simulink model "ADRC"  (R2024b)
settings: Solver=VariableStepAuto  StartTime=0.0  StopTime=40  FixedStep=0.001  RelTol=1e-3  EnableMultiTasking=on
settings Model: TunableVars=PP,PI,PD  TunableVarsStorageClass=ExportedGlobal,ExportedGlobal,ImportedExtern  TunableVarsTypeQualifier=const,const,const  Creator=yuy  LastModifiedBy=17989
settings SolverCC: AlgebraicLoopSolver=TrustRegion
settings DataIOCC: LimitDataPoints=on  SaveFormat=Array  ReturnWorkspaceOutputs=off
settings OptimizationCC: DefaultParameterBehavior=Inlined  LifeSpan=inf
settings DebuggingCC: AlgebraicLoopMsg=none  UnconnectedInputMsg=warning  UnconnectedOutputMsg=warning  UnconnectedLineMsg=warning  SFUnexpectedBacktrackingDiag=warning  SFNoUnconditionalDefaultTransitionDiag=warning  SFExecutionAtInitializationDiag=none  ArithmeticOperatorsInVariantConditions=warning
settings HardwareCC: ProdBitPerPointer=32  ProdBitPerSizeT=32  ProdBitPerPtrDiffT=32  ProdLargestAtomicFloat=None  ProdIntDivRoundTo=Undefined  ProdEndianess=Unspecified  ProdWordSize=32  ProdHWDeviceType=32-bit Generic
settings ModelReferenceCC: EnableRefExpFcnMdlSchedulingChecks=on  PropagateSignalLabelsOutOfModel=off
settings SFSimCC: SimUseLocalCustomCode=off  CustomCodeUndefinedFunction=UseInterfaceOnly
settings RTWCC: GenCodeOnly=on  PackageGeneratedCodeAndArtifacts=on  PackageName=ADRC  RTWUseLocalCustomCode=off  Toolchain=Microsoft Visual C++ 2017 v15.0 | nmake (64-bit Windows)  GPUComputeCapability=3.5
settings CodeAppCC: StateflowObjectComments=on
settings GRTTargetCC: TargetLangStandard=C89/C90 (ANSI)
settings ConfigComp: CovMetricSettings=dw  CovSaveCumulativeToWorkspaceVar=on  CovSaveSingleToWorkspaceVar=on  CovExternalEMLEnable=off  CovSFcnEnable=off

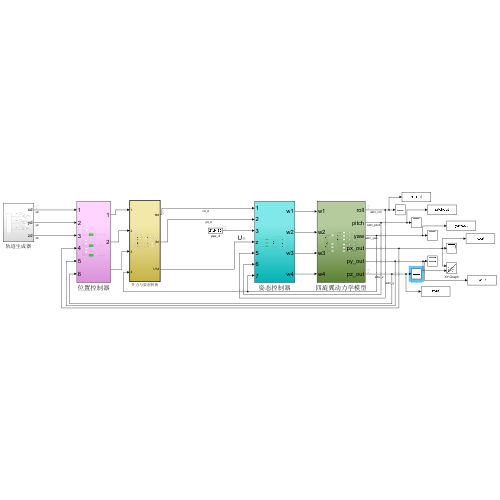
[thumbnail: Simulink's stored preview of the top-level diagram]
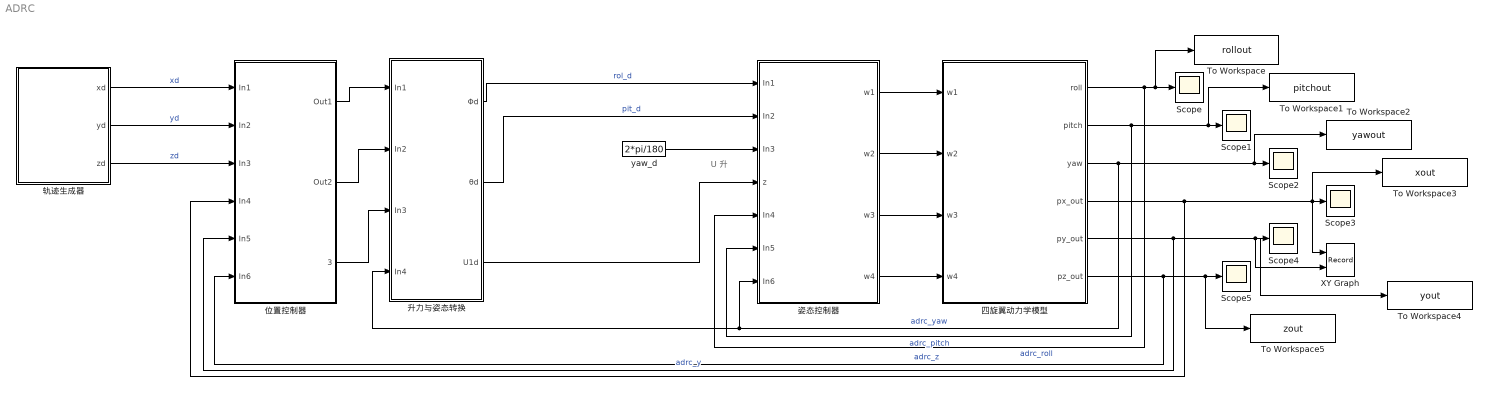
== system ADRC ==
  note: U 升
  Scope{,1..5} (6 alike) : Scope
  To Workspace : ToWorkspace  VariableName=rollout  SampleTime=-1
  To Workspace1 : ToWorkspace  VariableName=pitchout  SampleTime=-1
  To Workspace2 : ToWorkspace  VariableName=yawout  SampleTime=-1
  To Workspace3 : ToWorkspace  VariableName=xout  SampleTime=-1
  To Workspace4 : ToWorkspace  VariableName=yout  SampleTime=-1
  To Workspace5 : ToWorkspace  VariableName=zout  SampleTime=-1
  XY Graph : Record  FileSettingsInternal="{\"entries\":[{\"content\":{\"excelSettings\":{\"content\":{},\"type\":\"Streamout.ExcelSettings\"}},\"type\":\"Streamout.FileSettingStorage\",\"uuid\":\"\"}],\"packageUris\":[\"http:\\/\\/schema.mathworks.com\\/mf0\\/streamout_blocks\\/R2020a\"],\"version\":\"1.0\"}"  Layout=[1 1]  SignalsInternal="{\"entries\":[{\"content\":{\"signals\":[{\"content\":{\"blockPath\":[],\"dimensions\":[1],\"domain\":\"\",\"lineColor\":\"#a2142f\",\"lineWidth\":2,\"port\":1,\"sid\":[\"\"],\"signalID\":1,\"signalName\":\"四旋翼动力学模型:4\"},\"type\":\"RecordBlkView.Signal\",\"uuid\":\"\"},{\"content\":{\"blockPath\":[],\"dimensions\":[1],\"domain\":\"\",\"lineColor\":\"#139fff\",\"lineWidth\":2,\"port\":2,\"sid\":[\"\"],\"signalID\":2,\"signalName\":\"adrc_y\"},\"type\":\"RecordBlkView.Signal\",\"uuid\":\"\"}]},\"type\":\"RecordBlkView.InputSignals\",\"uuid\":\"\"}],\"packageUris\":[\"http:\\/\\/schema.mathworks.com\\/mf0\\/streamout_blocks\\/R2020a\"],\"version\":\"1.0\"}"  VisualizationBindings="{\"xyplotplugin\":{\"info\":[{\"series\":[],\"subplotID\":1}]}}"  CompatibilityTag=XY  st=-1
  yaw_d : Constant  Value=2*pi/180
  位置控制器 : Subsystem
  升力与姿态转换 : Subsystem  TreatAsAtomicUnit=on
  四旋翼动力学模型 : Subsystem
  姿态控制器 : Subsystem
  轨迹生成器 : Subsystem
  wires:
  四旋翼动力学模型/4(px_out) -> To Workspace3/1, XY Graph/1, Scope3/1, 位置控制器/4(In4)
  四旋翼动力学模型/5(py_out) -> To Workspace4/1, XY Graph/2, Scope4/1, 位置控制器/5(In5)  "adrc_y"
  四旋翼动力学模型/6(pz_out) -> To Workspace5/1, Scope5/1, 位置控制器/6(In6)  "adrc_z"
  四旋翼动力学模型/1(roll) -> To Workspace/1, Scope/1, 姿态控制器/5(In4)  "adrc_roll"
  姿态控制器/1(w1) -> 四旋翼动力学模型/1(w1)
  姿态控制器/2(w2) -> 四旋翼动力学模型/2(w2)
  姿态控制器/3(w3) -> 四旋翼动力学模型/3(w3)
  四旋翼动力学模型/3(yaw) -> To Workspace2/1, Scope2/1, 姿态控制器/7(In6), 升力与姿态转换/4(In4)  "adrc_yaw"
  姿态控制器/4(w4) -> 四旋翼动力学模型/4(w4)
  升力与姿态转换/1(Φd) -> 姿态控制器/1(In1)  "rol_d"
  升力与姿态转换/2(θd) -> 姿态控制器/2(In2)  "pit_d"
  四旋翼动力学模型/2(pitch) -> To Workspace1/1, Scope1/1, 姿态控制器/6(In5)  "adrc_pitch"
  位置控制器/1(Out1) -> 升力与姿态转换/1(In1)
  位置控制器/2(Out2) -> 升力与姿态转换/2(In2)
  位置控制器/3(" ") -> 升力与姿态转换/3(In3)
  轨迹生成器/1(xd) -> 位置控制器/1(In1)  "xd"
  轨迹生成器/3(zd) -> 位置控制器/3(In3)  "zd"
  轨迹生成器/2(yd) -> 位置控制器/2(In2)  "yd"
  yaw_d/1 -> 姿态控制器/3(In3)
  升力与姿态转换/3(U1d) -> 姿态控制器/4(z)

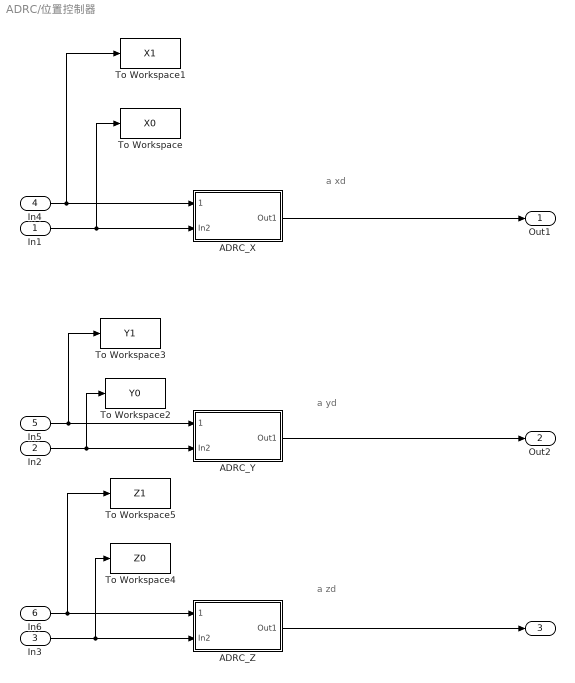
== system ADRC/位置控制器 ==
  note: a zd
  note: a yd
  note: a xd
  In1 : Inport
  In2 : Inport  Port=2
  In3 : Inport  Port=3
  In4 : Inport  Port=4
  In5 : Inport  Port=5
  In6 : Inport  Port=6
  "ADRC_X " : Subsystem
  ADRC_Y : Subsystem
  "ADRC_Z " : Subsystem
  To Workspace : ToWorkspace  VariableName=X0  SampleTime=-1
      settings: Save2DSignal=2-D array (concatenate along first dimension)
  To Workspace1 : ToWorkspace  VariableName=X1  SampleTime=-1
      settings: Save2DSignal=2-D array (concatenate along first dimension)
  To Workspace2 : ToWorkspace  VariableName=Y0  SampleTime=-1
      settings: Save2DSignal=2-D array (concatenate along first dimension)
  To Workspace3 : ToWorkspace  VariableName=Y1  SampleTime=-1
      settings: Save2DSignal=2-D array (concatenate along first dimension)
  To Workspace4 : ToWorkspace  VariableName=Z0  SampleTime=-1
      settings: Save2DSignal=2-D array (concatenate along first dimension)
  To Workspace5 : ToWorkspace  VariableName=Z1  SampleTime=-1
      settings: Save2DSignal=2-D array (concatenate along first dimension)
  Out1 : Outport
  Out2 : Outport  Port=2
  " " : Outport  Port=3
  wires:
  In3/1 -> To Workspace4/1, "ADRC_Z "/2(In2)
  In6/1 -> To Workspace5/1, "ADRC_Z "/1(" ")
  In5/1 -> To Workspace3/1, ADRC_Y/1(" ")
  In2/1 -> ADRC_Y/2(In2), To Workspace2/1
  In1/1 -> To Workspace/1, "ADRC_X "/2(In2)
  In4/1 -> To Workspace1/1, "ADRC_X "/1(" ")
  "ADRC_X "/1(Out1) -> Out1/1
  ADRC_Y/1(Out1) -> Out2/1
  "ADRC_Z "/1(Out1) -> " "/1

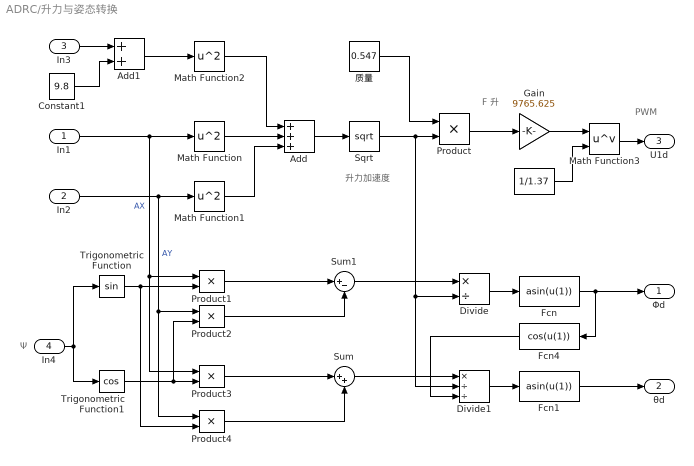
== system ADRC/升力与姿态转换 ==
  note: PWM
  note: 升力加速度
  note: F 升
  note: Ψ
  In1 : Inport
  In2 : Inport  Port=2
  In3 : Inport  Port=3
  In4 : Inport  Port=4
  " " : Constant  Value=1/1.37
  Add : Sum  Inputs=+++
  Add1 : Sum
  Constant1 : Constant  Value=9.8
  Divide : Product  Inputs=*/
  Divide1 : Product  Inputs=*//
  Fcn : Fcn  Expr=asin(u(1))
  Fcn1 : Fcn  Expr=asin(u(1))
  Fcn4 : Fcn  Expr=cos(u(1))
  Gain : Gain  Gain=9765.625
  Math Function3 : Math  Operator=pow  SignedPower=on
  Math Function : Math  Operator=square  SignedPower=on
  Math Function1 : Math  Operator=square  SignedPower=on
  Math Function2 : Math  Operator=square  SignedPower=on
  Product{,1..4} (5 alike) : Product  RndMeth=Zero
  Sqrt : Sqrt
  Sum : Sum  Inputs=|++
  Sum1 : Sum  Inputs=|+-
  Trigonometric Function : Trigonometry
  Trigonometric Function1 : Trigonometry  Operator=cos
  质量 : Constant  Value=0.547
  Φd : Outport
  θd : Outport  Port=2
  U1d : Outport  Port=3
  wires:
  In2/1 -> Math Function1/1, Product2/1, Product4/1  "AY"
  Add/1 -> Sqrt/1
  Sqrt/1 -> Divide1/2, Divide/2, Product/2
  质量/1 -> Product/1
  Fcn/1 -> Φd/1, Fcn4/1
  Divide/1 -> Fcn/1
  Constant1/1 -> Add1/2
  In3/1 -> Add1/1
  Add1/1 -> Math Function2/1
  Fcn1/1 -> θd/1
  Divide1/1 -> Fcn1/1
  In4/1 -> Trigonometric Function/1, Trigonometric Function1/1
  Trigonometric Function/1 -> Product1/2, Product4/2
  Trigonometric Function1/1 -> Product2/2, Product3/2
  Product1/1 -> Sum1/1
  Product2/1 -> Sum1/2
  Sum1/1 -> Divide/1
  In1/1 -> Math Function/1, Product1/1, Product3/1  "AX"
  Product3/1 -> Sum/1
  Product4/1 -> Sum/2
  Sum/1 -> Divide1/1
  Fcn4/1 -> Divide1/3
  Gain/1 -> Math Function3/1
  " "/1 -> Math Function3/2
  Product/1 -> Gain/1
  Math Function3/1 -> U1d/1
  Math Function2/1 -> Add/1
  Math Function/1 -> Add/2
  Math Function1/1 -> Add/3

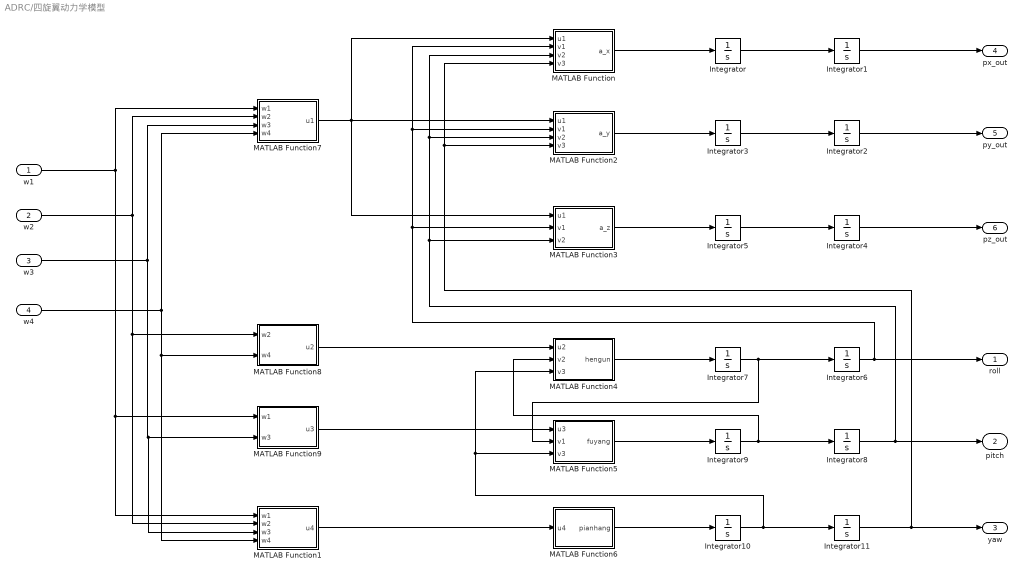
== system ADRC/四旋翼动力学模型 ==
  w1 : Inport
  w2 : Inport  Port=2
  w3 : Inport  Port=3
  w4 : Inport  Port=4
  Integrator{,1..11} (12 alike) : Integrator
  MATLAB Function : MATLAB Function  TreatAsAtomicUnit=on
  MATLAB Function1 : MATLAB Function  TreatAsAtomicUnit=on
  MATLAB Function2 : MATLAB Function  TreatAsAtomicUnit=on
  MATLAB Function3 : MATLAB Function  TreatAsAtomicUnit=on
  MATLAB Function4 : MATLAB Function  TreatAsAtomicUnit=on
  MATLAB Function5 : MATLAB Function  TreatAsAtomicUnit=on
  MATLAB Function6 : MATLAB Function  TreatAsAtomicUnit=on
  MATLAB Function7 : MATLAB Function  TreatAsAtomicUnit=on
  MATLAB Function8 : MATLAB Function  TreatAsAtomicUnit=on
  MATLAB Function9 : MATLAB Function  TreatAsAtomicUnit=on
  roll : Outport
  pitch : Outport  Port=2
  yaw : Outport  Port=3
  px_out : Outport  Port=4
  py_out : Outport  Port=5
  pz_out : Outport  Port=6
  wires:
  w4/1 -> MATLAB Function7/4(w4), MATLAB Function1/4(w4), MATLAB Function8/2(w4)
  w3/1 -> MATLAB Function1/3(w3), MATLAB Function9/2(w3), MATLAB Function7/3(w3)
  Integrator/1 -> Integrator1/1
  MATLAB Function2/1(a_y) -> Integrator3/1
  Integrator3/1 -> Integrator2/1
  MATLAB Function3/1(a_z) -> Integrator5/1
  Integrator5/1 -> Integrator4/1
  MATLAB Function7/1(u1) -> MATLAB Function/1(u1), MATLAB Function3/1(u1), MATLAB Function2/1(u1)
  MATLAB Function1/1(u4) -> MATLAB Function6/1(u4)
  MATLAB Function9/1(u3) -> MATLAB Function5/1(u3)
  MATLAB Function/1(a_x) -> Integrator/1
  MATLAB Function8/1(u2) -> MATLAB Function4/1(u2)
  MATLAB Function6/1(pianhang) -> Integrator10/1
  MATLAB Function4/1(hengun) -> Integrator7/1
  Integrator4/1 -> pz_out/1
  Integrator11/1 -> yaw/1, MATLAB Function2/4(v3), MATLAB Function/4(v3)
  w1/1 -> MATLAB Function1/1(w1), MATLAB Function9/1(w1), MATLAB Function7/1(w1)
  w2/1 -> MATLAB Function1/2(w2), MATLAB Function8/1(w2), MATLAB Function7/2(w2)
  Integrator7/1 -> MATLAB Function5/2(v1), Integrator6/1
  MATLAB Function5/1(fuyang) -> Integrator9/1
  Integrator2/1 -> py_out/1
  Integrator10/1 -> MATLAB Function4/3(v3), MATLAB Function5/3(v3), Integrator11/1
  Integrator8/1 -> pitch/1, MATLAB Function2/3(v2), MATLAB Function/3(v2), MATLAB Function3/3(v2)
  Integrator6/1 -> roll/1, MATLAB Function2/2(v1), MATLAB Function/2(v1), MATLAB Function3/2(v1)
  Integrator9/1 -> MATLAB Function4/2(v2), Integrator8/1
  Integrator1/1 -> px_out/1

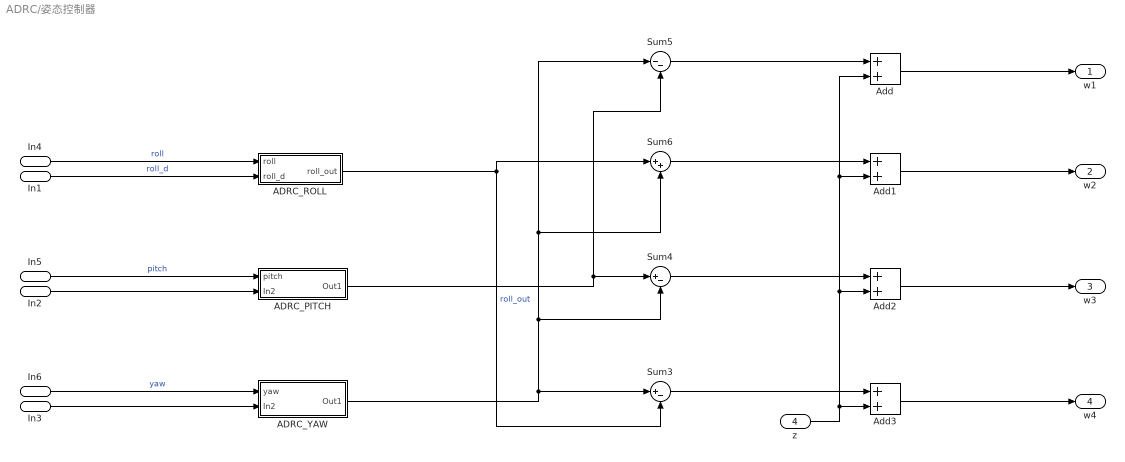
== system ADRC/姿态控制器 ==
  In1 : Inport
  In2 : Inport  Port=2
  In3 : Inport  Port=3
  z : Inport  Port=4
  In4 : Inport  Port=5
  In5 : Inport  Port=6
  In6 : Inport  Port=7
  "ADRC_PITCH " : Subsystem
  "ADRC_ROLL " : Subsystem
  ADRC_YAW : Subsystem
  Add{,1..3} (4 alike) : Sum
  Sum3 : Sum  Inputs=|+-
  Sum4 : Sum  Inputs=|+-
  Sum5 : Sum  Inputs=|--
  Sum6 : Sum  Inputs=|++
  w1 : Outport
  w2 : Outport  Port=2
  w3 : Outport  Port=3
  w4 : Outport  Port=4
  wires:
  Add2/1 -> w3/1
  Sum6/1 -> Add1/1
  Sum3/1 -> Add3/1
  Add1/1 -> w2/1
  Add3/1 -> w4/1
  Sum5/1 -> Add/1
  Add/1 -> w1/1
  Sum4/1 -> Add2/1
  "ADRC_ROLL "/1(roll_out) -> Sum6/1, Sum3/2  "roll_out"
  In4/1 -> "ADRC_ROLL "/1(roll)  "roll"
  In1/1 -> "ADRC_ROLL "/2(roll_d)  "roll_d"
  In5/1 -> "ADRC_PITCH "/1(pitch)  "pitch"
  In2/1 -> "ADRC_PITCH "/2(In2)
  In6/1 -> ADRC_YAW/1(yaw)  "yaw"
  In3/1 -> ADRC_YAW/2(In2)
  z/1 -> Add/2, Add1/2, Add2/2, Add3/2
  "ADRC_PITCH "/1(Out1) -> Sum5/2, Sum4/1
  ADRC_YAW/1(Out1) -> Sum4/2, Sum6/2, Sum5/1, Sum3/1

== system ADRC/轨迹生成器 ==
  note: Z d
  note: Yd
  note: Xd
  Manual Switch : ManualSwitch  CurrentSetting=0
  Manual Switch1 : ManualSwitch  CurrentSetting=0
  Manual Switch2 : ManualSwitch  CurrentSetting=0
  Step : Step  After=0.05  SampleTime=0
  Step1 : Step  Time=5  After=0.05  SampleTime=0
  Step2 : Step  Time=0  After=0.05  SampleTime=0
  Subsystem1 : Subsystem
  xd : Outport
  yd : Outport  Port=2
  zd : Outport  Port=3
  wires:
  Manual Switch/1 -> xd/1
  Subsystem1/1(Out1) -> Manual Switch/2  "expect:x"
  Step/1 -> Manual Switch/1
  Step1/1 -> Manual Switch1/1
  Manual Switch1/1 -> yd/1
  Subsystem1/2(Out2) -> Manual Switch1/2  "expect:y"
  Step2/1 -> Manual Switch2/1
  Manual Switch2/1 -> zd/1
  Subsystem1/3(Out3) -> Manual Switch2/2  "expect:z"

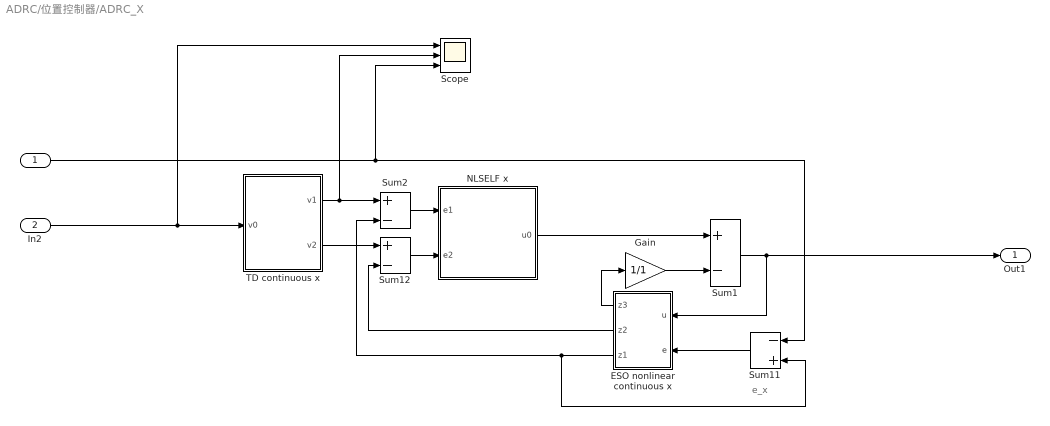
== system ADRC/位置控制器/ADRC_X  ==
  note: e_x
  " " : Inport
  In2 : Inport  Port=2
  ESO nonlinear continuous x : Subsystem
  Gain : Gain  Gain=1/1
  NLSELF x : Subsystem
  Scope : Scope  NumInputPorts=3
  Sum1 : Sum  Inputs=+-
  Sum11 : Sum  Inputs=-+
  Sum12 : Sum  Inputs=+-
  Sum2 : Sum  Inputs=+-
  TD continuous x : Subsystem
  Out1 : Outport
  wires:
  Sum1/1 -> Out1/1, ESO nonlinear continuous x/1(u)
  NLSELF x/1(u0) -> Sum1/1
  ESO nonlinear continuous x/3(z1) -> Sum2/2, Sum11/2
  ESO nonlinear continuous x/1(z3) -> Gain/1
  TD continuous x/1(v1) -> Scope/2, Sum2/1
  ESO nonlinear continuous x/2(z2) -> Sum12/2
  Gain/1 -> Sum1/2
  Sum11/1 -> ESO nonlinear continuous x/2(e)
  TD continuous x/2(v2) -> Sum12/1
  Sum2/1 -> NLSELF x/1(e1)
  Sum12/1 -> NLSELF x/2(e2)
  In2/1 -> Scope/1, TD continuous x/1(v0)
  " "/1 -> Scope/3, Sum11/1

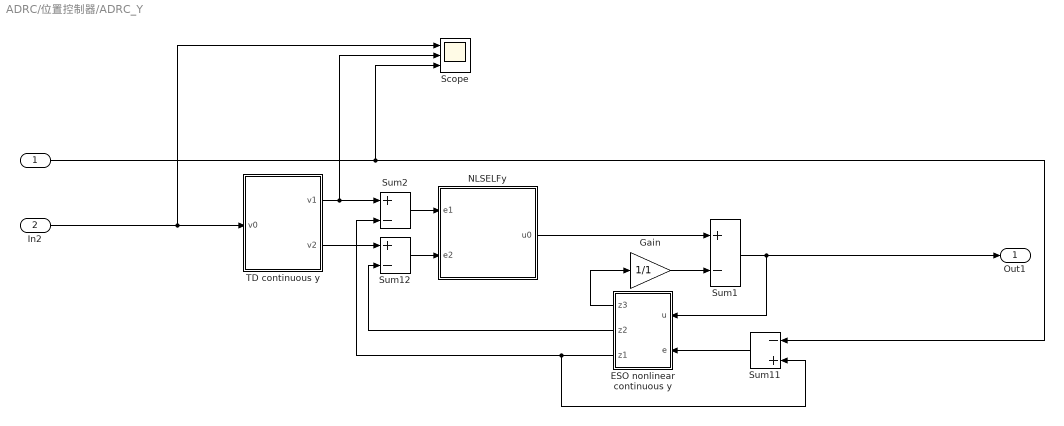
== system ADRC/位置控制器/ADRC_Y ==
  " " : Inport
  In2 : Inport  Port=2
  ESO nonlinear continuous y : Subsystem
  Gain : Gain  Gain=1/1
  NLSELFy : Subsystem
  Scope : Scope  NumInputPorts=3
  Sum1 : Sum  Inputs=+-
  Sum11 : Sum  Inputs=-+
  Sum12 : Sum  Inputs=+-
  Sum2 : Sum  Inputs=+-
  TD continuous y : Subsystem
  Out1 : Outport
  wires:
  Sum1/1 -> Out1/1, ESO nonlinear continuous y/1(u)
  NLSELFy/1(u0) -> Sum1/1
  ESO nonlinear continuous y/3(z1) -> Sum2/2, Sum11/2
  ESO nonlinear continuous y/1(z3) -> Gain/1
  TD continuous y/1(v1) -> Scope/2, Sum2/1
  ESO nonlinear continuous y/2(z2) -> Sum12/2
  Gain/1 -> Sum1/2
  Sum11/1 -> ESO nonlinear continuous y/2(e)
  TD continuous y/2(v2) -> Sum12/1
  Sum2/1 -> NLSELFy/1(e1)
  Sum12/1 -> NLSELFy/2(e2)
  In2/1 -> Scope/1, TD continuous y/1(v0)
  " "/1 -> Scope/3, Sum11/1

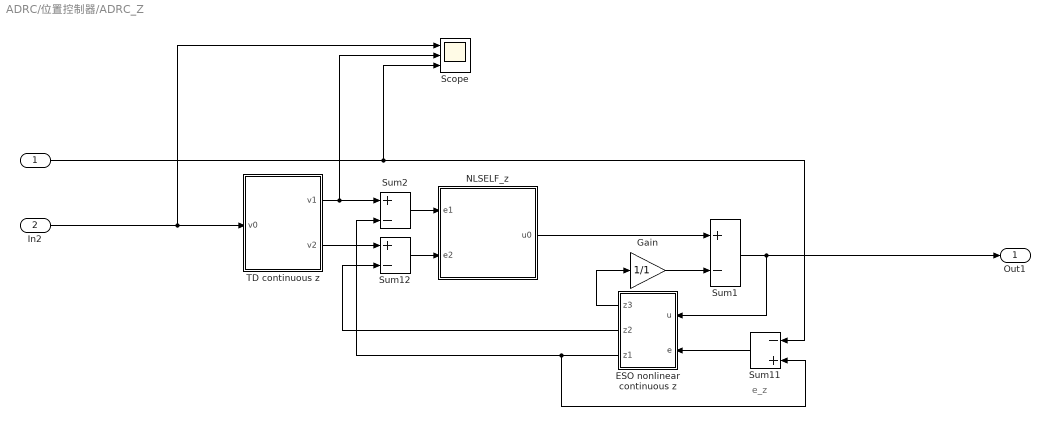
== system ADRC/位置控制器/ADRC_Z  ==
  note: e_z
  " " : Inport
  In2 : Inport  Port=2
  ESO nonlinear continuous z : Subsystem
  Gain : Gain  Gain=1/1
  NLSELF_z : Subsystem
  Scope : Scope  NumInputPorts=3
  Sum1 : Sum  Inputs=+-
  Sum11 : Sum  Inputs=-+
  Sum12 : Sum  Inputs=+-
  Sum2 : Sum  Inputs=+-
  TD continuous z : Subsystem
  Out1 : Outport
  wires:
  Sum1/1 -> Out1/1, ESO nonlinear continuous z/1(u)
  NLSELF_z/1(u0) -> Sum1/1
  ESO nonlinear continuous z/3(z1) -> Sum2/2, Sum11/2
  ESO nonlinear continuous z/1(z3) -> Gain/1
  TD continuous z/1(v1) -> Scope/2, Sum2/1
  ESO nonlinear continuous z/2(z2) -> Sum12/2
  Gain/1 -> Sum1/2
  Sum11/1 -> ESO nonlinear continuous z/2(e)
  TD continuous z/2(v2) -> Sum12/1
  Sum2/1 -> NLSELF_z/1(e1)
  Sum12/1 -> NLSELF_z/2(e2)
  In2/1 -> Scope/1, TD continuous z/1(v0)
  " "/1 -> Scope/3, Sum11/1

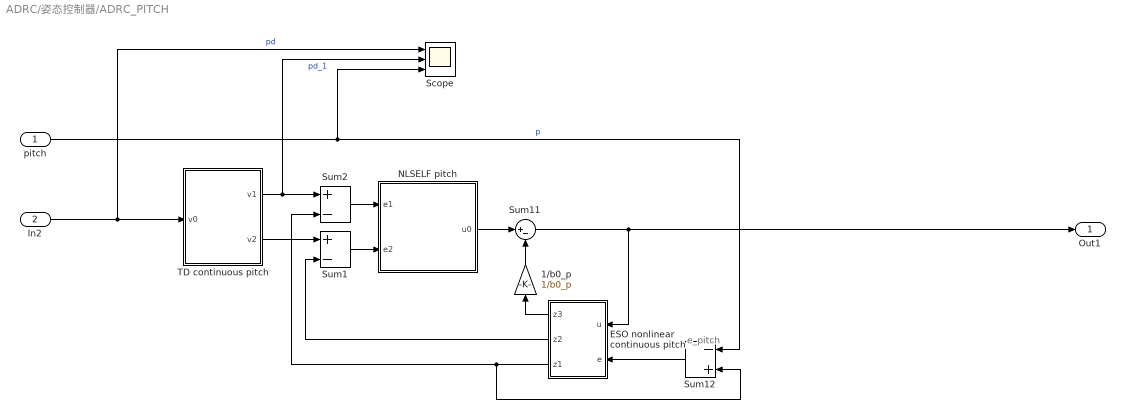
== system ADRC/姿态控制器/ADRC_PITCH  ==
  note: e_pitch
  pitch : Inport
  In2 : Inport  Port=2
  1/b0_p : Gain  Gain=1/b0_p  mask{b0_p=0.08}
  ESO nonlinear continuous pitch : Subsystem
  NLSELF pitch : Subsystem
  Scope : Scope  NumInputPorts=3
  Sum1 : Sum  Inputs=+-
  Sum11 : Sum  Inputs=|+-
  Sum12 : Sum  Inputs=-+
  Sum2 : Sum  Inputs=+-
  TD continuous pitch : Subsystem
  Out1 : Outport
  wires:
  TD continuous pitch/1(v1) -> Scope/2, Sum2/1  "pd_1"
  Sum1/1 -> NLSELF pitch/2(e2)
  Sum11/1 -> Out1/1, ESO nonlinear continuous pitch/1(u)
  TD continuous pitch/2(v2) -> Sum1/1
  1/b0_p/1 -> Sum11/2
  ESO nonlinear continuous pitch/3(z1) -> Sum2/2, Sum12/2
  ESO nonlinear continuous pitch/1(z3) -> 1/b0_p/1
  Sum12/1 -> ESO nonlinear continuous pitch/2(e)
  NLSELF pitch/1(u0) -> Sum11/1
  ESO nonlinear continuous pitch/2(z2) -> Sum1/2
  Sum2/1 -> NLSELF pitch/1(e1)
  In2/1 -> Scope/1, TD continuous pitch/1(v0)  "pd"
  pitch/1 -> Scope/3, Sum12/1  "p"

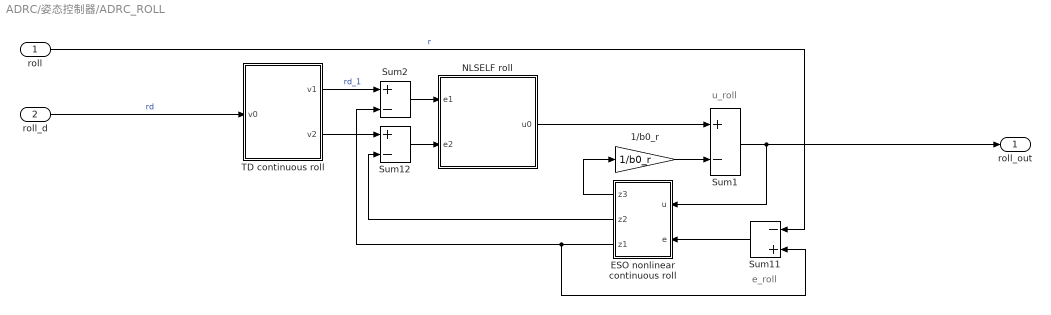
== system ADRC/姿态控制器/ADRC_ROLL  ==
  note: u_roll
  note: e_roll
  roll : Inport
  roll_d : Inport  Port=2
  1/b0_r : Gain  Gain=1/b0_r  mask{b0_r=0.08}
  ESO nonlinear continuous roll : Subsystem
  NLSELF roll : Subsystem
  Sum1 : Sum  Inputs=+-
  Sum11 : Sum  Inputs=-+
  Sum12 : Sum  Inputs=+-
  Sum2 : Sum  Inputs=+-
  TD continuous roll : Subsystem
  roll_out : Outport
  wires:
  Sum1/1 -> roll_out/1, ESO nonlinear continuous roll/1(u)
  NLSELF roll/1(u0) -> Sum1/1
  ESO nonlinear continuous roll/3(z1) -> Sum2/2, Sum11/2
  ESO nonlinear continuous roll/1(z3) -> 1/b0_r/1
  TD continuous roll/1(v1) -> Sum2/1  "rd_1"
  ESO nonlinear continuous roll/2(z2) -> Sum12/2
  1/b0_r/1 -> Sum1/2
  Sum11/1 -> ESO nonlinear continuous roll/2(e)
  TD continuous roll/2(v2) -> Sum12/1
  Sum2/1 -> NLSELF roll/1(e1)
  Sum12/1 -> NLSELF roll/2(e2)
  roll_d/1 -> TD continuous roll/1(v0)  "rd"
  roll/1 -> Sum11/1  "r"

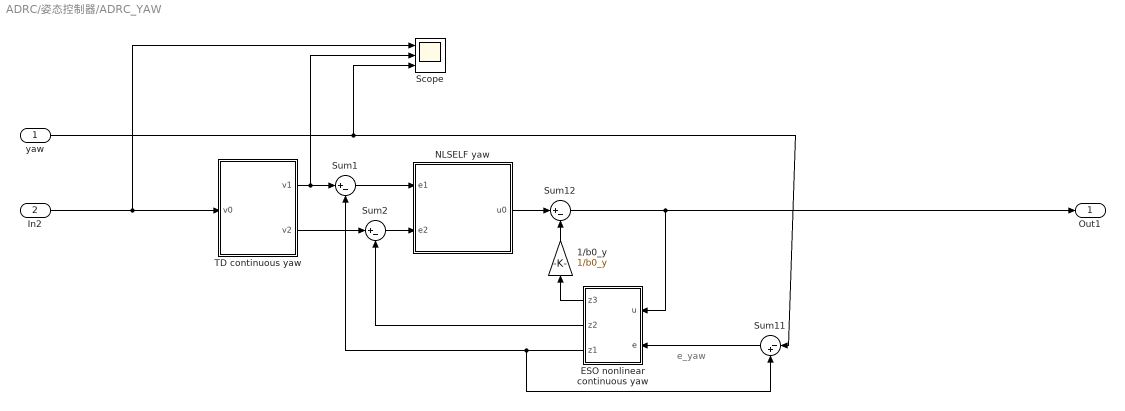
== system ADRC/姿态控制器/ADRC_YAW ==
  note: e_yaw
  yaw : Inport
  In2 : Inport  Port=2
  1/b0_y : Gain  Gain=1/b0_y  mask{b0_y=0.013}
  ESO nonlinear continuous yaw : Subsystem
  NLSELF yaw : Subsystem
  Scope : Scope  NumInputPorts=3
  Sum1 : Sum  Inputs=|+-
  Sum11 : Sum  Inputs=|-+
  Sum12 : Sum  Inputs=|+-
  Sum2 : Sum  Inputs=|+-
  TD continuous yaw : Subsystem
  Out1 : Outport
  wires:
  TD continuous yaw/1(v1) -> Scope/2, Sum1/1
  Sum2/1 -> NLSELF yaw/2(e2)
  ESO nonlinear continuous yaw/2(z2) -> Sum2/2
  ESO nonlinear continuous yaw/3(z1) -> Sum1/2, Sum11/2
  1/b0_y/1 -> Sum12/2
  Sum11/1 -> ESO nonlinear continuous yaw/2(e)
  Sum1/1 -> NLSELF yaw/1(e1)
  Sum12/1 -> Out1/1, ESO nonlinear continuous yaw/1(u)
  TD continuous yaw/2(v2) -> Sum2/1
  ESO nonlinear continuous yaw/1(z3) -> 1/b0_y/1
  NLSELF yaw/1(u0) -> Sum12/1
  In2/1 -> Scope/1, TD continuous yaw/1(v0)
  yaw/1 -> Scope/3, Sum11/1

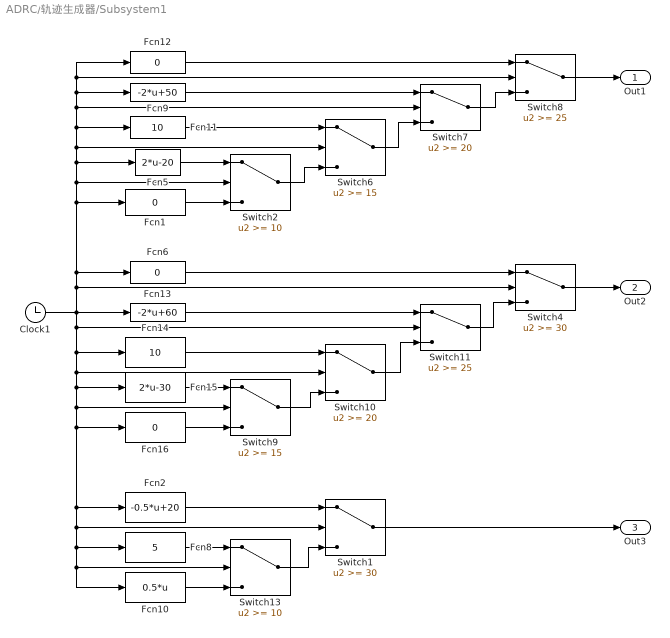
== system ADRC/轨迹生成器/Subsystem1 ==
  Clock1 : Clock
  Fcn{1,6,12,16} (4 alike) : Fcn  Expr=0
  Fcn10 : Fcn  Expr=0.5*u
  Fcn11 : Fcn  Expr=10
  Fcn13 : Fcn  Expr=-2*u+60
  Fcn14 : Fcn  Expr=10
  Fcn15 : Fcn  Expr=2*u-30
  Fcn2 : Fcn  Expr=-0.5*u+20
  Fcn5 : Fcn  Expr=2*u-20
  Fcn8 : Fcn  Expr=5
  Fcn9 : Fcn  Expr=-2*u+50
  Switch1 : Switch  Threshold=30  SaturateOnIntegerOverflow=off  InputSameDT=off
  Switch10 : Switch  Threshold=20  SaturateOnIntegerOverflow=off  InputSameDT=off
  Switch11 : Switch  Threshold=25  SaturateOnIntegerOverflow=off  InputSameDT=off
  Switch13 : Switch  Threshold=10  SaturateOnIntegerOverflow=off  InputSameDT=off
  Switch2 : Switch  Threshold=10  SaturateOnIntegerOverflow=off  InputSameDT=off
  Switch4 : Switch  Threshold=30  SaturateOnIntegerOverflow=off  InputSameDT=off
  Switch6 : Switch  Threshold=15  SaturateOnIntegerOverflow=off  InputSameDT=off
  Switch7 : Switch  Threshold=20  SaturateOnIntegerOverflow=off  InputSameDT=off
  Switch8 : Switch  Threshold=25  SaturateOnIntegerOverflow=off  InputSameDT=off
  Switch9 : Switch  Threshold=15  SaturateOnIntegerOverflow=off  InputSameDT=off
  Out1 : Outport
  Out2 : Outport  Port=2
  Out3 : Outport  Port=3
  wires:
  Fcn12/1 -> Switch8/1
  Switch7/1 -> Switch8/3
  Fcn9/1 -> Switch7/1
  Switch2/1 -> Switch6/3
  Switch6/1 -> Switch7/3
  Fcn11/1 -> Switch6/1
  Switch8/1 -> Out1/1
  Fcn14/1 -> Switch10/1
  Fcn16/1 -> Switch9/3
  Switch10/1 -> Switch11/3
  Switch9/1 -> Switch10/3
  Fcn15/1 -> Switch9/1
  Fcn13/1 -> Switch11/1
  Fcn1/1 -> Switch2/3
  Fcn5/1 -> Switch2/1
  Switch11/1 -> Switch4/3
  Fcn6/1 -> Switch4/1
  Switch4/1 -> Out2/1
  Clock1/1 -> Fcn1/1, Fcn9/1, Switch8/2, Fcn12/1, Switch7/2, Fcn11/1, Switch6/2, Fcn5/1, Switch2/2, Fcn6/1, Switch4/2, Fcn13/1, Switch11/2, Switch10/2, Fcn15/1, Switch9/2, Fcn16/1, Switch1/2, Fcn10/1, Switch13/2, Fcn8/1, Fcn2/1, Fcn14/1
  Fcn8/1 -> Switch13/1
  Fcn10/1 -> Switch13/3
  Fcn2/1 -> Switch1/1
  Switch1/1 -> Out3/1
  Switch13/1 -> Switch1/3

== system ADRC/位置控制器/ADRC_X /ESO nonlinear continuous x ==
  u : Inport
  e : Inport  Port=2
  Integrator : Integrator
  Integrator1 : Integrator
  Integrator2 : Integrator
  MATLAB Function : MATLAB Function  TreatAsAtomicUnit=on
  z3 : Outport
  z2 : Outport  Port=2
  z1 : Outport  Port=3
  wires:
  Integrator/1 -> z1/1
  MATLAB Function/1(dz1) -> Integrator/1
  MATLAB Function/2(dz2) -> Integrator1/1
  Integrator1/1 -> MATLAB Function/3(z2), z2/1
  MATLAB Function/3(dz3) -> Integrator2/1
  u/1 -> MATLAB Function/1(u)
  e/1 -> MATLAB Function/2(e)
  Integrator2/1 -> MATLAB Function/4(z3), z3/1

== system ADRC/位置控制器/ADRC_X /NLSELF x ==
  e1 : Inport
  e2 : Inport  Port=2
  MATLAB Function : MATLAB Function  TreatAsAtomicUnit=on
  u0 : Outport
  wires:
  MATLAB Function/1(u0) -> u0/1
  e1/1 -> MATLAB Function/1(e1)
  e2/1 -> MATLAB Function/2(e2)

== system ADRC/位置控制器/ADRC_X /TD continuous x ==
  v0 : Inport
  Integrator : Integrator
  Integrator1 : Integrator
  MATLAB Function : MATLAB Function  TreatAsAtomicUnit=on
  v1 : Outport
  v2 : Outport  Port=2
  wires:
  v0/1 -> MATLAB Function/1(v0)
  MATLAB Function/1(dv1) -> Integrator/1
  Integrator/1 -> MATLAB Function/2(v1), v1/1
  Integrator1/1 -> MATLAB Function/3(v2), v2/1
  MATLAB Function/2(dv2) -> Integrator1/1

== system ADRC/位置控制器/ADRC_Y/ESO nonlinear continuous y ==
  u : Inport
  e : Inport  Port=2
  Integrator : Integrator
  Integrator1 : Integrator
  Integrator2 : Integrator
  MATLAB Function : MATLAB Function  TreatAsAtomicUnit=on
  z3 : Outport
  z2 : Outport  Port=2
  z1 : Outport  Port=3
  wires:
  Integrator/1 -> z1/1
  MATLAB Function/1(dz1) -> Integrator/1
  MATLAB Function/2(dz2) -> Integrator1/1
  Integrator1/1 -> MATLAB Function/3(z2), z2/1
  MATLAB Function/3(dz3) -> Integrator2/1
  u/1 -> MATLAB Function/1(u)
  e/1 -> MATLAB Function/2(e)
  Integrator2/1 -> MATLAB Function/4(z3), z3/1

== system ADRC/位置控制器/ADRC_Y/NLSELFy ==
  e1 : Inport
  e2 : Inport  Port=2
  MATLAB Function : MATLAB Function  TreatAsAtomicUnit=on
  u0 : Outport
  wires:
  MATLAB Function/1(u0) -> u0/1
  e1/1 -> MATLAB Function/1(e1)
  e2/1 -> MATLAB Function/2(e2)

== system ADRC/位置控制器/ADRC_Y/TD continuous y ==
  v0 : Inport
  Integrator : Integrator
  Integrator1 : Integrator
  MATLAB Function : MATLAB Function  TreatAsAtomicUnit=on
  v1 : Outport
  v2 : Outport  Port=2
  wires:
  v0/1 -> MATLAB Function/1(v0)
  MATLAB Function/1(dv1) -> Integrator/1
  Integrator/1 -> MATLAB Function/2(v1), v1/1
  Integrator1/1 -> MATLAB Function/3(v2), v2/1
  MATLAB Function/2(dv2) -> Integrator1/1

== system ADRC/位置控制器/ADRC_Z /ESO nonlinear continuous z ==
  u : Inport
  e : Inport  Port=2
  Integrator : Integrator
  Integrator1 : Integrator
  Integrator2 : Integrator
  MATLAB Function : MATLAB Function  TreatAsAtomicUnit=on
  z3 : Outport
  z2 : Outport  Port=2
  z1 : Outport  Port=3
  wires:
  Integrator/1 -> z1/1
  MATLAB Function/1(dz1) -> Integrator/1
  MATLAB Function/2(dz2) -> Integrator1/1
  Integrator1/1 -> MATLAB Function/3(z2), z2/1
  MATLAB Function/3(dz3) -> Integrator2/1
  u/1 -> MATLAB Function/1(u)
  e/1 -> MATLAB Function/2(e)
  Integrator2/1 -> MATLAB Function/4(z3), z3/1

== system ADRC/位置控制器/ADRC_Z /NLSELF_z ==
  e1 : Inport
  e2 : Inport  Port=2
  MATLAB Function : MATLAB Function  TreatAsAtomicUnit=on
  u0 : Outport
  wires:
  MATLAB Function/1(u0) -> u0/1
  e1/1 -> MATLAB Function/1(e1)
  e2/1 -> MATLAB Function/2(e2)

== system ADRC/位置控制器/ADRC_Z /TD continuous z ==
  v0 : Inport
  Integrator : Integrator
  Integrator1 : Integrator
  MATLAB Function : MATLAB Function  TreatAsAtomicUnit=on
  v1 : Outport
  v2 : Outport  Port=2
  wires:
  v0/1 -> MATLAB Function/1(v0)
  MATLAB Function/1(dv1) -> Integrator/1
  Integrator/1 -> MATLAB Function/2(v1), v1/1
  Integrator1/1 -> MATLAB Function/3(v2), v2/1
  MATLAB Function/2(dv2) -> Integrator1/1

== system ADRC/姿态控制器/ADRC_PITCH /ESO nonlinear continuous pitch ==
  u : Inport
  e : Inport  Port=2
  Integrator : Integrator
  Integrator1 : Integrator
  Integrator2 : Integrator
  MATLAB Function : MATLAB Function  TreatAsAtomicUnit=on
  z3 : Outport
  z2 : Outport  Port=2
  z1 : Outport  Port=3
  wires:
  Integrator/1 -> z1/1
  MATLAB Function/1(dz1) -> Integrator/1
  MATLAB Function/2(dz2) -> Integrator1/1
  Integrator1/1 -> MATLAB Function/3(z2), z2/1
  MATLAB Function/3(dz3) -> Integrator2/1
  Integrator2/1 -> MATLAB Function/4(z3), z3/1
  u/1 -> MATLAB Function/1(u)
  e/1 -> MATLAB Function/2(e)

== system ADRC/姿态控制器/ADRC_PITCH /NLSELF pitch ==
  e1 : Inport
  e2 : Inport  Port=2
  MATLAB Function : MATLAB Function  TreatAsAtomicUnit=on
  u0 : Outport
  wires:
  MATLAB Function/1(u0) -> u0/1
  e1/1 -> MATLAB Function/1(e1)
  e2/1 -> MATLAB Function/2(e2)

== system ADRC/姿态控制器/ADRC_PITCH /TD continuous pitch ==
  v0 : Inport
  Integrator : Integrator
  Integrator1 : Integrator
  MATLAB Function : MATLAB Function  TreatAsAtomicUnit=on
  v1 : Outport
  v2 : Outport  Port=2
  wires:
  v0/1 -> MATLAB Function/1(v0)
  MATLAB Function/1(dv1) -> Integrator/1
  Integrator/1 -> MATLAB Function/2(v1), v1/1
  Integrator1/1 -> MATLAB Function/3(v2), v2/1
  MATLAB Function/2(dv2) -> Integrator1/1

== system ADRC/姿态控制器/ADRC_ROLL /ESO nonlinear continuous roll ==
  u : Inport
  e : Inport  Port=2
  Integrator : Integrator
  Integrator1 : Integrator
  Integrator2 : Integrator
  MATLAB Function : MATLAB Function  TreatAsAtomicUnit=on
  z3 : Outport
  z2 : Outport  Port=2
  z1 : Outport  Port=3
  wires:
  Integrator/1 -> z1/1
  MATLAB Function/1(dz1) -> Integrator/1
  MATLAB Function/2(dz2) -> Integrator1/1
  Integrator1/1 -> MATLAB Function/3(z2), z2/1
  MATLAB Function/3(dz3) -> Integrator2/1
  u/1 -> MATLAB Function/1(u)
  e/1 -> MATLAB Function/2(e)
  Integrator2/1 -> MATLAB Function/4(z3), z3/1

== system ADRC/姿态控制器/ADRC_ROLL /NLSELF roll ==
  e1 : Inport
  e2 : Inport  Port=2
  MATLAB Function : MATLAB Function  TreatAsAtomicUnit=on
  u0 : Outport
  wires:
  MATLAB Function/1(u0) -> u0/1
  e1/1 -> MATLAB Function/1(e1)
  e2/1 -> MATLAB Function/2(e2)

== system ADRC/姿态控制器/ADRC_ROLL /TD continuous roll ==
  v0 : Inport
  Integrator : Integrator
  Integrator1 : Integrator
  MATLAB Function : MATLAB Function  TreatAsAtomicUnit=on
  v1 : Outport
  v2 : Outport  Port=2
  wires:
  v0/1 -> MATLAB Function/1(v0)
  MATLAB Function/1(dv1) -> Integrator/1
  Integrator/1 -> MATLAB Function/2(v1), v1/1
  Integrator1/1 -> MATLAB Function/3(v2), v2/1
  MATLAB Function/2(dv2) -> Integrator1/1

== system ADRC/姿态控制器/ADRC_YAW/ESO nonlinear continuous yaw ==
  u : Inport
  e : Inport  Port=2
  Integrator : Integrator
  Integrator1 : Integrator
  Integrator2 : Integrator
  MATLAB Function : MATLAB Function  TreatAsAtomicUnit=on
  z3 : Outport
  z2 : Outport  Port=2
  z1 : Outport  Port=3
  wires:
  Integrator/1 -> z1/1
  MATLAB Function/1(dz1) -> Integrator/1
  MATLAB Function/2(dz2) -> Integrator1/1
  Integrator1/1 -> MATLAB Function/3(z2), z2/1
  MATLAB Function/3(dz3) -> Integrator2/1
  u/1 -> MATLAB Function/1(u)
  e/1 -> MATLAB Function/2(e)
  Integrator2/1 -> MATLAB Function/4(z3), z3/1

== system ADRC/姿态控制器/ADRC_YAW/NLSELF yaw ==
  e1 : Inport
  e2 : Inport  Port=2
  MATLAB Function : MATLAB Function  TreatAsAtomicUnit=on
  u0 : Outport
  wires:
  MATLAB Function/1(u0) -> u0/1
  e1/1 -> MATLAB Function/1(e1)
  e2/1 -> MATLAB Function/2(e2)

== system ADRC/姿态控制器/ADRC_YAW/TD continuous yaw ==
  v0 : Inport
  Integrator : Integrator
  Integrator1 : Integrator
  MATLAB Function : MATLAB Function  TreatAsAtomicUnit=on
  v1 : Outport
  v2 : Outport  Port=2
  wires:
  v0/1 -> MATLAB Function/1(v0)
  MATLAB Function/1(dv1) -> Integrator/1
  Integrator/1 -> MATLAB Function/2(v1), v1/1
  Integrator1/1 -> MATLAB Function/3(v2), v2/1
  MATLAB Function/2(dv2) -> Integrator1/1

== matlab function ADRC/姿态控制器/ADRC_ROLL /ESO nonlinear continuous roll/MATLAB Function ==
  data: u input; dz1 output; e input; dz2 output; dz3 output; z2 input; z3 input
function [dz1,dz2,dz3] = fcn(u,e,z2, z3)
%#连续形式的扩张状态观测器(ESO)

%% 参数赋值
beta01_r = 30;     % 可调参数
beta02_r = 300;     % 可调参数
beta03_r = 1000;   % 可调参数
a1 = 0.75;         % 可调参数
a2 = 0.5;          % 可调参数
a3 = 0.25;         % 可调参数
delta = 3;     % 线性段的区间长度
b0_r = 0.08;       % 决定补偿强弱的“补偿因子”

dz1 = z2 - beta01_r * fal(e, a1, delta);
dz2 = z3 - beta02_r * fal(e, a2, delta) + b0_r * u;
dz3 = - beta03_r * fal(e, a3, delta);

== matlab function ADRC/姿态控制器/ADRC_ROLL /NLSELF roll/MATLAB Function ==
  data: e1 input; u0 output; e2 input
function u0 = fcn(e1,e2)
%#非线性状态误差反馈律(NLSEF)

%% 参数赋值
beta1_r = 1000;   % 可调参数
beta2_r = 2700;   % 可调参数
delta_r = 5;     % 线性段的区间长度
a1 = 0.5;        % 可调参数
a2 = 0.05;       % 可调参数
%% 一种采用fal()函数组合的NLSEF算法
u0 = beta1_r * fal(e1, a1, delta_r) + beta2_r * fal(e2, a2, delta_r);

== matlab function ADRC/四旋翼动力学模型/MATLAB Function1 ==
  data: w1 input; u4 output; w2 input; w3 input; w4 input
function u4 = fcn(w1,w2,w3,w4)
%#codegen

u4 = 1.20*10^-6*(w2^1.25+w4^1.25-w1^1.25-w3^1.25);

== matlab function ADRC/姿态控制器/ADRC_ROLL /TD continuous roll/MATLAB Function ==
  data: v0 input; dv1 output; dv2 output; v1 input; v2 input
function [dv1, dv2] = fcn(v0, v1, v2)
%连续型跟踪微分器TD
%% 参数赋值
h0 = 0.01;            % 滤波因子
omega_r = 180;         % 决定跟踪快慢的参数
%% 连续形式的跟踪微分器算法
dv1 = v2;
dv2 = fst(v1-v0, v2, omega_r, h0);

== matlab function ADRC/姿态控制器/ADRC_PITCH /ESO nonlinear continuous pitch/MATLAB Function ==
  data: u input; dz1 output; e input; dz2 output; dz3 output; z2 input; z3 input
function [dz1,dz2,dz3] = fcn(u,e,z2, z3)
%#连续形式的扩张状态观测器(ESO)

%% 参数赋值
beta01_p = 30;     % 可调参数
beta02_p = 300;     % 可调参数
beta03_p = 1000;   % 可调参数
a1 = 0.75;         % 可调参数
a2 = 0.5;          % 可调参数
a3 = 0.25;         % 可调参数
delta = 3;     % 线性段的区间长度
b0_p = 0.08;       % 决定补偿强弱的“补偿因子”

dz1 = z2 - beta01_p * fal(e, a1, delta);
dz2 = z3 - beta02_p * fal(e, a2, delta) + b0_p * u;
dz3 = - beta03_p * fal(e, a3, delta);

== matlab function ADRC/姿态控制器/ADRC_PITCH /NLSELF pitch/MATLAB Function ==
  data: e1 input; u0 output; e2 input
function u0 = fcn(e1,e2)
%#非线性状态误差反馈律(NLSEF)

%% 参数赋值
beta1_p = 1000;   % 可调参数
beta2_p = 2700;   % 可调参数
delta_p = 5;     % 线性段的区间长度
a1 = 0.5;        % 可调参数
a2 = 0.05;       % 可调参数
%% 一种采用fal()函数组合的NLSEF算法
u0 = beta1_p * fal(e1, a1, delta_p) + beta2_p * fal(e2, a2, delta_p);

== matlab function ADRC/姿态控制器/ADRC_PITCH /TD continuous pitch/MATLAB Function ==
  data: v0 input; dv1 output; dv2 output; v1 input; v2 input
function [dv1, dv2] = fcn(v0, v1, v2)
%连续型跟踪微分器TD
%% 参数赋值
h0 = 0.01;            % 滤波因子
omega_p = 180;         % 决定跟踪快慢的参数
%% 连续形式的跟踪微分器算法
dv1 = v2;
dv2 = fst(v1-v0, v2, omega_p, h0);

== matlab function ADRC/姿态控制器/ADRC_YAW/ESO nonlinear continuous yaw/MATLAB Function ==
  data: dz1 output; dz2 output; dz3 output; u input; e input; z2 input; z3 input
function [dz1,dz2,dz3] = fcn(u,e,z2, z3)
%#连续形式的扩张状态观测器(ESO)

%% 参数赋值
beta01_y = 30;     % 可调参数
beta02_y = 300;     % 可调参数
beta03_y = 1000;   % 可调参数
a1 = 0.75;         % 可调参数
a2 = 0.5;          % 可调参数
a3 = 0.25;         % 可调参数
delta = 5;     % 线性段的区间长度
b0_y = 0.013;       % 决定补偿强弱的“补偿因子”

dz1 = z2 - beta01_y * fal(e, a1, delta);
dz2 = z3 - beta02_y * fal(e, a2, delta) + b0_y * u;
dz3 = - beta03_y * fal(e, a3, delta);

== matlab function ADRC/姿态控制器/ADRC_YAW/NLSELF yaw/MATLAB Function ==
  data: e1 input; u0 output; e2 input
function u0 = fcn(e1,e2)
%#非线性状态误差反馈律(NLSEF)

%% 参数赋值
beta1_y =8000;   % 可调参数
beta2_y =12000;   % 可调参数
delta_y = 6;     % 线性段的区间长度
a1 = 0.5;        % 可调参数
a2 = 0.05;       % 可调参数
%% 一种采用fal()函数组合的NLSEF算法
u0 = beta1_y * fal(e1, a1, delta_y) + beta2_y * fal(e2, a2, delta_y);

== matlab function ADRC/姿态控制器/ADRC_YAW/TD continuous yaw/MATLAB Function ==
  data: v0 input; dv1 output; dv2 output; v1 input; v2 input
function [dv1, dv2] = fcn(v0, v1, v2)
%连续型跟踪微分器TD
%% 参数赋值
h0 = 0.008;            % 滤波因子
omega_y = 100;         % 决定跟踪快慢的参数
%% 连续形式的跟踪微分器算法
dv1 = v2;
dv2 = fst(v1-v0, v2, omega_y, h0);

== matlab function ADRC/位置控制器/ADRC_X /ESO nonlinear continuous x/MATLAB Function ==
  data: u input; dz1 output; e input; dz2 output; dz3 output; z2 input; z3 input
function [dz1,dz2,dz3] = fcn(u,e,z2, z3)
%#连续形式的扩张状态观测器(ESO)

%% 参数赋值
beta01_x = 30;     % 可调参数
beta02_x = 300;     % 可调参数
beta03_x = 1000;   % 可调参数
a1 = 0.75;         % 可调参数
a2 = 0.5;          % 可调参数
a3 = 0.25;         % 可调参数
delta = 2;     % 线性段的区间长度
b0_x = 1;       % 决定补偿强弱的“补偿因子”

dz1 = z2 - beta01_x * fal(e, a1, delta);
dz2 = z3 - beta02_x * fal(e, a2, delta) + b0_x * u;
dz3 = - beta03_x * fal(e, a3, delta);

== matlab function ADRC/位置控制器/ADRC_X /NLSELF x/MATLAB Function ==
  data: e1 input; u0 output; e2 input
function u0 = fcn(e1,e2)
%#非线性状态误差反馈律(NLSEF)

%% 参数赋值
beta1_x =2;   % 可调参数
beta2_x = 24;   % 可调参数
delta_x = 2;     % 线性段的区间长度
a1 = 0.5;        % 可调参数
a2 = 0.05;       % 可调参数
%% 一种采用fal()函数组合的NLSEF算法
u0 = beta1_x * fal(e1, a1, delta_x) + beta2_x * fal(e2, a2, delta_x);

== matlab function ADRC/位置控制器/ADRC_X /TD continuous x/MATLAB Function ==
  data: v0 input; dv1 output; dv2 output; v1 input; v2 input
function [dv1, dv2] = fcn(v0, v1, v2)
%连续型跟踪微分器TD
%% 参数赋值
h0 = 0.01;            % 滤波因子
omega_x =300;         % 决定跟踪快慢的参数
%% 连续形式的跟踪微分器算法
dv1 = v2;
dv2 = fst(v1-v0, v2, omega_x, h0);

== matlab function ADRC/四旋翼动力学模型/MATLAB Function ==
  data: u1 input; a_x output; v1 input; v2 input; v3 input
function a_x = fcn(u1,v1,v2,v3)
%#codegen

a_x = (u1/0.547)*(cos(v1)*sin(v2)*cos(v3)+sin(v1)*sin(v3));

== matlab function ADRC/位置控制器/ADRC_Y/ESO nonlinear continuous y/MATLAB Function ==
  data: u input; dz1 output; e input; dz2 output; dz3 output; z2 input; z3 input
function [dz1,dz2,dz3] = fcn(u,e,z2, z3)
%#连续形式的扩张状态观测器(ESO)

%% 参数赋值
beta01_y = 30;     % 可调参数
beta02_y = 300;     % 可调参数
beta03_y = 1000;   % 可调参数
a1 = 0.75;         % 可调参数
a2 = 0.5;          % 可调参数
a3 = 0.25;         % 可调参数
delta = 2;     % 线性段的区间长度
b0_yy = 1;       % 决定补偿强弱的“补偿因子”

dz1 = z2 - beta01_y * fal(e, a1, delta);
dz2 = z3 - beta02_y * fal(e, a2, delta) + b0_yy * u;
dz3 = - beta03_y * fal(e, a3, delta);

== matlab function ADRC/位置控制器/ADRC_Y/NLSELFy/MATLAB Function ==
  data: e1 input; u0 output; e2 input
function u0 = fcn(e1,e2)
%#非线性状态误差反馈律(NLSEF)

%% 参数赋值
beta1_y =2;   % 可调参数
beta2_y = 24;   % 可调参数
delta_y = 2;     % 线性段的区间长度
a1 = 0.5;        % 可调参数
a2 = 0.05;       % 可调参数
%% 一种采用fal()函数组合的NLSEF算法
u0 = beta1_y * fal(e1, a1, delta_y) + beta2_y * fal(e2, a2, delta_y);

== matlab function ADRC/位置控制器/ADRC_Y/TD continuous y/MATLAB Function ==
  data: v0 input; dv1 output; dv2 output; v1 input; v2 input
function [dv1, dv2] = fcn(v0, v1, v2)
%连续型跟踪微分器TD
%% 参数赋值
h0 = 0.01;            % 滤波因子
omega_y =300;         % 决定跟踪快慢的参数
%% 连续形式的跟踪微分器算法
dv1 = v2;
dv2 = fst(v1-v0, v2, omega_y, h0);

== matlab function ADRC/位置控制器/ADRC_Z /ESO nonlinear continuous z/MATLAB Function ==
  data: u input; dz1 output; e input; dz2 output; dz3 output; z2 input; z3 input
function [dz1,dz2,dz3] = fcn(u,e,z2, z3)
%#连续形式的扩张状态观测器(ESO)

%% 参数赋值
beta01_z = 30;     % 可调参数
beta02_z = 300;     % 可调参数
beta03_z = 1000;   % 可调参数
a1 = 0.75;         % 可调参数
a2 = 0.5;          % 可调参数
a3 = 0.25;         % 可调参数
delta = 3;     % 线性段的区间长度
b0_z = 1;       % 决定补偿强弱的“补偿因子”

dz1 = z2 - beta01_z * fal(e, a1, delta);
dz2 = z3 - beta02_z * fal(e, a2, delta) + b0_z * u;
dz3 = - beta03_z * fal(e, a3, delta);

== matlab function ADRC/位置控制器/ADRC_Z /NLSELF_z/MATLAB Function ==
  data: e1 input; u0 output; e2 input
function u0 = fcn(e1,e2)
%#非线性状态误差反馈律(NLSEF)

%% 参数赋值
beta1_z = 10;   % 可调参数
beta2_z = 30;   % 可调参数
delta_z = 3;     % 线性段的区间长度
a1 = 0.5;        % 可调参数
a2 = 0.05;       % 可调参数
%% 一种采用fal()函数组合的NLSEF算法
u0 = beta1_z * fal(e1, a1, delta_z) + beta2_z * fal(e2, a2, delta_z);

== matlab function ADRC/位置控制器/ADRC_Z /TD continuous z/MATLAB Function ==
  data: v0 input; dv1 output; dv2 output; v1 input; v2 input
function [dv1, dv2] = fcn(v0, v1, v2)
%连续型跟踪微分器TD
%% 参数赋值
h0 = 0.01;            % 滤波因子
omega_z = 180;         % 决定跟踪快慢的参数
%% 连续形式的跟踪微分器算法
dv1 = v2;
dv2 = fst(v1-v0, v2, omega_z, h0);

== matlab function ADRC/四旋翼动力学模型/MATLAB Function2 ==
  data: u1 input; a_y output; v1 input; v2 input; v3 input
function a_y = fcn(u1,v1,v2,v3)
%#codegen

a_y = (u1/0.547)*(cos(v1)*sin(v2)*sin(v3)-sin(v1)*cos(v3));

== matlab function ADRC/四旋翼动力学模型/MATLAB Function3 ==
  data: u1 input; a_z output; v1 input; v2 input
function a_z = fcn(u1,v1,v2)
%#codegen

a_z = (u1/0.547)*cos(v1)*cos(v2)-9.8;

== matlab function ADRC/四旋翼动力学模型/MATLAB Function4 ==
  data: u2 input; hengun output; v2 input; v3 input
function hengun = fcn(u2,v2,v3)
%#codegen

hengun = (u2/0.0033)-v2*v3*(0.0025/0.0033);

== matlab function ADRC/四旋翼动力学模型/MATLAB Function5 ==
  data: u3 input; fuyang output; v1 input; v3 input
function fuyang = fcn(u3,v1,v3)
%#codegen

fuyang = (u3/0.0033)+v1*v3*(0.0025/0.0033);

== matlab function ADRC/四旋翼动力学模型/MATLAB Function6 ==
  data: u4 input; pianhang output
function pianhang = fcn(u4)
%#codegen

pianhang = u4/0.0033;

== matlab function ADRC/四旋翼动力学模型/MATLAB Function7 ==
  data: w1 input; u1 output; w2 input; w3 input; w4 input
function u1 = fcn(w1,w2,w3,w4)
%#codegen

u1=2.56*10^-5*(w1^1.37+w2^1.37+w3^1.37+w4^1.37);

== matlab function ADRC/四旋翼动力学模型/MATLAB Function8 ==
  data: w2 input; u2 output; w4 input
function u2 = fcn(w2,w4)
%#codegen

u2 =2.56*10^-5*(w2^1.37-w4^1.37)*0.2;

== matlab function ADRC/四旋翼动力学模型/MATLAB Function9 ==
  data: w1 input; u3 output; w3 input
function u3 = fcn(w1,w3)
%#codegen

u3 =2.56*10^-5*(w3^1.37-w1^1.37)*0.2;
